simulink model "sfunction"  (R2024a)
settings: Solver=VariableStepAuto  StartTime=0.0  StopTime=10  RelTol=1e-3
libraries: fuzblock x3
settings Model: Creator=ericliu  LastModifiedBy=Eason

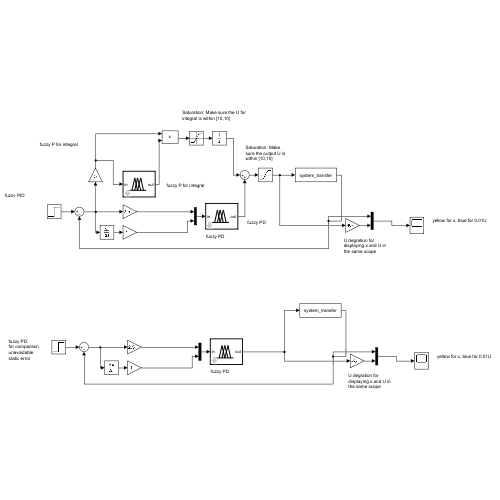
[thumbnail: Simulink's stored preview of the top-level diagram]
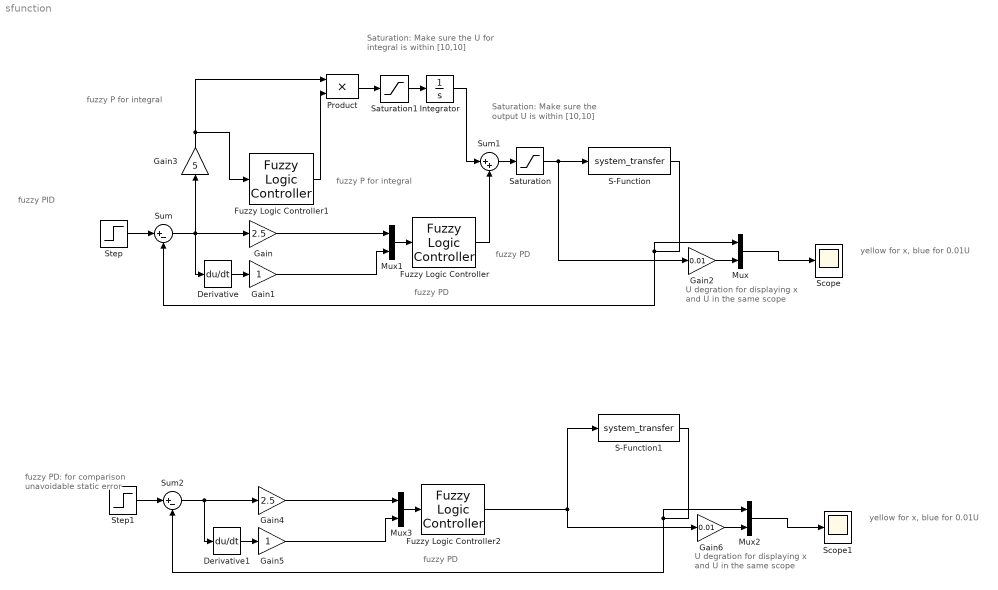
== system sfunction ==
  note: fuzzy PD:
      | for comparison
      | unavoidable static error
  note: fuzzy PID
  note: fuzzy PD
  note: U degration for displaying x and U in the same scope
  note: fuzzy PD
  note: fuzzy P for integral
  note: Saturation: Make sure the U for integral is within [10,10]
  note: Saturation: Make sure the output U is within [10,10]
  note: fuzzy P for integral
  note: yellow for x, blue for 0.01U
  note: U degration for displaying x and U in the same scope
  note: yellow for x, blue for 0.01U
  note: fuzzy PD
  Derivative : Derivative
  Derivative1 : Derivative
  Fuzzy Logic Controller : fuzblock/Fuzzy Logic  Controller  FIS='fuzzy.fis'  OutputSampleNumber=101  DataType=double  FuzzifiedInputs=off  RuleFiringStrengths=off  RuleOutputs=off  AggregatedOutputs=off  SimulateUsing=Interpreted execution  OutOfRangeInputValueMessage=warning  NoRuleFiredMessage=warning  EmptyOutputFuzzySetMessage=warning
  Fuzzy Logic Controller1 : fuzblock/Fuzzy Logic  Controller  FIS='fuzzy_p.fis'  OutputSampleNumber=101  DataType=double  FuzzifiedInputs=off  RuleFiringStrengths=off  RuleOutputs=off  AggregatedOutputs=off  SimulateUsing=Interpreted execution  OutOfRangeInputValueMessage=warning  NoRuleFiredMessage=warning  EmptyOutputFuzzySetMessage=warning
  Fuzzy Logic Controller2 : fuzblock/Fuzzy Logic  Controller  FIS='fuzzy.fis'  OutputSampleNumber=101  DataType=double  FuzzifiedInputs=off  RuleFiringStrengths=off  RuleOutputs=off  AggregatedOutputs=off  SimulateUsing=Interpreted execution  OutOfRangeInputValueMessage=warning  NoRuleFiredMessage=warning  EmptyOutputFuzzySetMessage=warning
  Gain : Gain  Gain=2.5
  Gain1 : Gain
  Gain2 : Gain  Gain=0.01
  Gain3 : Gain  Gain=5
  Gain4 : Gain  Gain=2.5
  Gain5 : Gain
  Gain6 : Gain  Gain=0.01
  Integrator : Integrator
  Mux{,1..3} (4 alike) : Mux  Inputs=2
  Product : Product
  S-Function : S-Function  FunctionName=system_transfer  SFunctionDeploymentMode=off  EnableBusSupport=off
  S-Function1 : S-Function  FunctionName=system_transfer  SFunctionDeploymentMode=off  EnableBusSupport=off
  Saturation : Saturate  UpperLimit=10  LowerLimit=-10
  Saturation1 : Saturate  UpperLimit=10  LowerLimit=-10
  Scope : Scope
  Scope1 : Scope
  Step : Step  Time=0  After=0.05  SampleTime=0
  Step1 : Step  Time=0  After=0.05  SampleTime=0
  Sum : Sum  Inputs=|+-
  Sum1 : Sum  Inputs=|++
  Sum2 : Sum  Inputs=|+-
  wires:
  Step/1 -> Sum/1
  Mux/1 -> Scope/1
  Derivative/1 -> Gain1/1
  Sum/1 -> Gain3/1, Derivative/1, Gain/1
  Mux1/1 -> Fuzzy Logic Controller/1
  Fuzzy Logic Controller/1 -> Sum1/2
  S-Function/1 -> Mux/1, Sum/2
  Gain/1 -> Mux1/1
  Gain1/1 -> Mux1/2
  Gain2/1 -> Mux/2
  Fuzzy Logic Controller1/1 -> Product/2
  Sum1/1 -> Saturation/1
  Saturation/1 -> Gain2/1, S-Function/1
  Gain3/1 -> Fuzzy Logic Controller1/1, Product/1
  Product/1 -> Saturation1/1
  Integrator/1 -> Sum1/1
  Saturation1/1 -> Integrator/1
  S-Function1/1 -> Mux2/1, Sum2/2
  Fuzzy Logic Controller2/1 -> S-Function1/1, Gain6/1
  Gain4/1 -> Mux3/1
  Mux3/1 -> Fuzzy Logic Controller2/1
  Derivative1/1 -> Gain5/1
  Sum2/1 -> Derivative1/1, Gain4/1
  Gain6/1 -> Mux2/2
  Mux2/1 -> Scope1/1
  Step1/1 -> Sum2/1
  Gain5/1 -> Mux3/2
